simulink subsystem "EncoderAJvel"  (R2023b)
settings: Solver=VariableStepAuto  StartTime=0.0  StopTime=10.0  RelTol=1e-3
libraries: arduinosensorlib x2
settings Model: Creator=johan  LastModifiedBy=Carlos

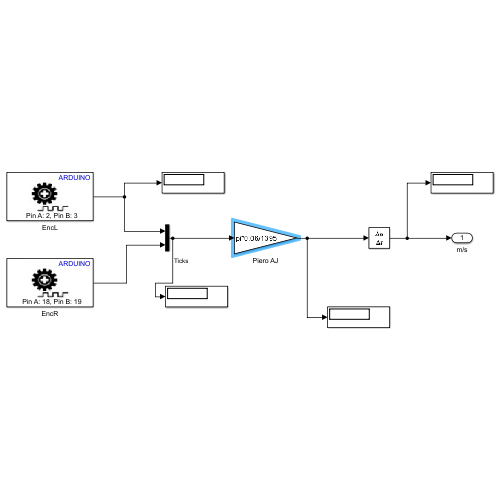
[thumbnail: Simulink's stored preview of the top-level diagram]
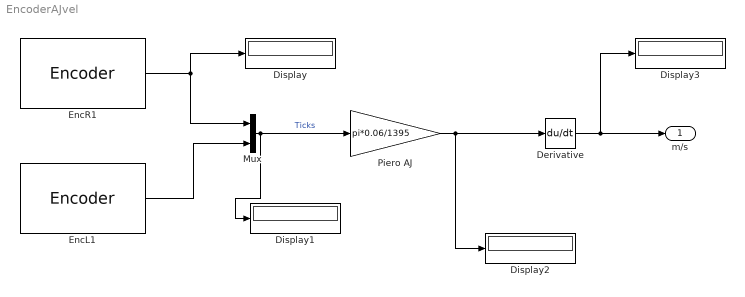
== system EncoderAJvel ==
  Derivative : Derivative
  Display{,1..3} (4 alike) : Display
  EncL1 : arduinosensorlib/Encoder  InputA=2  InputB=3  Mode=No reset  SampleTime=-1
  EncR1 : arduinosensorlib/Encoder  InputA=18  InputB=19  Mode=No reset  SampleTime=-1
  Mux : Mux  Inputs=2
  Piero AJ : Gain  Gain=pi*0.06/1395  OutDataTypeStr=double
  m/s : Outport  OutDataTypeStr=double
  wires:
  EncL1/1 -> Mux/2
  Derivative/1 -> m/s/1, Display3/1
  EncR1/1 -> Display/1, Mux/1
  Mux/1 -> Display1/1, Piero AJ/1  "Ticks"
  Piero AJ/1 -> Display2/1, Derivative/1
